simulink model "damper"  (R2020a)
settings: Solver=VariableStepAuto  StartTime=0.0  StopTime=10.0  RelTol=1e-3
undefined symbols (not defined in the file): sigbuilder_block
settings Model: Creator=Batukhan  LastModifiedBy=Batukhan

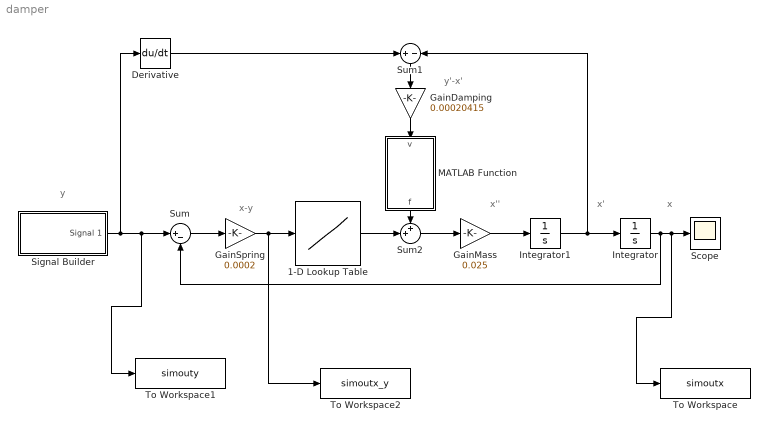
== system damper ==
  note: x
  note: y'-x'
  note: x'
  note: x''
  note: x-y
  note: y
  1-D Lookup Table : Lookup_n-D  NumberOfTableDimensions=1  BreakpointsForDimension1=[-0.5 -0.1 0 0.1 0.5]  Table=[-4500 500 0 500 4500]  InternalRulePriority=Speed  RndMeth=Simplest  InputSameDT=on
  Derivative : Derivative
  GainDamping : Gain  Gain=0.00020415
  GainMass : Gain  Gain=0.025
  GainSpring : Gain  Gain=0.0002
  Integrator : Integrator
  Integrator1 : Integrator
  MATLAB Function : MATLAB Function  TreatAsAtomicUnit=on
  Scope : Scope
  Signal Builder : Subsystem  Tag=STV Subsys  LoadFcn=sigbuilder_block('load');  StartFcn=sigbuilder_block('start');  StopFcn=sigbuilder_block('stop');  ClipboardFcn=sigbuilder_block('clipboard');  mask(Sigbuilder block){tuvar=[0:10]}
      mask help: Simulink:masks:SigbuilderBlock_MD
      mask init:
      | if ~strcmp(get_param(bdroot(gcbh),'SimulationStatus'),'stopped') tuvar = sigbuilder_block('maskInit'); end
      settings: CopyFcn=sigbuilder_block('copy');  DeleteFcn=sigbuilder_block('delete');  ModelCloseFcn=sigbuilder_block('modelClose');  PreSaveFcn=sigbuilder_block('preSave');  PauseFcn=sigbuilder_block('pause');  ContinueFcn=sigbuilder_block('continue');  NameChangeFcn=sigbuilder_block('namechange');  OpenFcn=sigbuilder_block('open',[785.25 170.25 550.5 399.75 ]);  CloseFcn=sigbuilder_block('close');
      mask Display: plot(0, 0, 100, 100,[2, 2, 32, 32, 2], [68, 8, 8, 68, 68],[32, 2], [38, 38], [32, 19, 2],[53, 60, 44], [32, 17, 17, 2],[16, 16, 31, 31]);txt = getActiveGroup(gcbh);text(2, 100, txt,'verticalAlignment', 'top');
  Sum : Sum  Inputs=|+-
  Sum1 : Sum  Inputs=+-
  Sum2 : Sum  Inputs=++|
  To Workspace : ToWorkspace  VariableName=simoutx  SampleTime=-1
      settings: Save2DSignal=2-D array (concatenate along first dimension)
  To Workspace1 : ToWorkspace  VariableName=simouty  SampleTime=-1
      settings: Save2DSignal=2-D array (concatenate along first dimension)
  To Workspace2 : ToWorkspace  VariableName=simoutx_y  SampleTime=-1
      settings: Save2DSignal=2-D array (concatenate along first dimension)
  wires:
  Signal Builder/1(Signal 1) -> To Workspace1/1, Sum/1, Derivative/1
  Derivative/1 -> Sum1/1
  Sum/1 -> GainSpring/1
  1-D Lookup Table/1 -> Sum2/2
  MATLAB Function/1(f) -> Sum2/1
  Sum2/1 -> GainMass/1
  GainMass/1 -> Integrator1/1
  Integrator1/1 -> Sum1/2, Integrator/1
  Integrator/1 -> To Workspace/1, Scope/1, Sum/2
  GainSpring/1 -> To Workspace2/1, 1-D Lookup Table/1
  Sum1/1 -> GainDamping/1
  GainDamping/1 -> MATLAB Function/1(v)

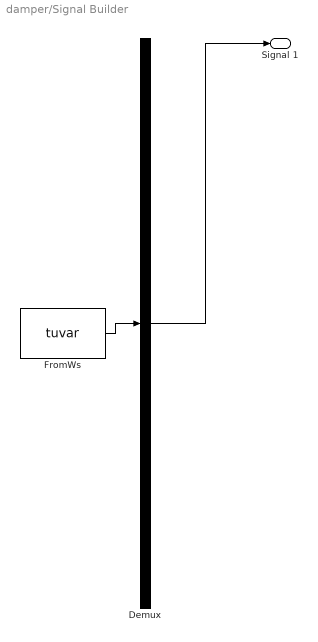
== system damper/Signal Builder ==
  Demux : Demux  Tag=STV Demux  Outputs=1
      settings: DisplayOption=none
  FromWs : FromWorkspace  Tag=STV FromWs  VariableName=tuvar
      SigBuilderData=|
      | common.afterFinalStr = 'Extrapolate'
      | common.sampleTime = 0
      | dataSet.timeRange = [0 10]
      | dataSet.name = 'Group 1'
      | sbobj.Groups.Name = 'Group 1'
      | sbobj.Groups.Signals.Name = 'Signal 1'
      | sbobj.Groups.Signals.XData = [0 0.1 3 3.16 6 10]
      | sbobj.Groups.Signals.YData = [0 0.2 0.2 0.002 0 0]
      | sbobj.Groups.TimeRange = [0 10]
  Signal 1 : Outport  Tag=STV Outport
  wires:
  Demux/1 -> Signal 1/1
  FromWs/1 -> Demux/1

== matlab function damper/MATLAB Function ==
  data: v input; f output
function f = damper(v)

if v <= 0
    f = -800*(abs(v)).^0.6;
else
    f = 200*v.^0.6;
end
